simulink model "Integrated_Model"  (R2018a)
settings: Solver=VariableStepAuto  StartTime=0.0  StopTime=500  RelTol=1e-3
undefined symbols (not defined in the file or in its folder): sgn
libraries: simulink x5
settings Model: Creator=梁鑫  LastModifiedBy=梁鑫

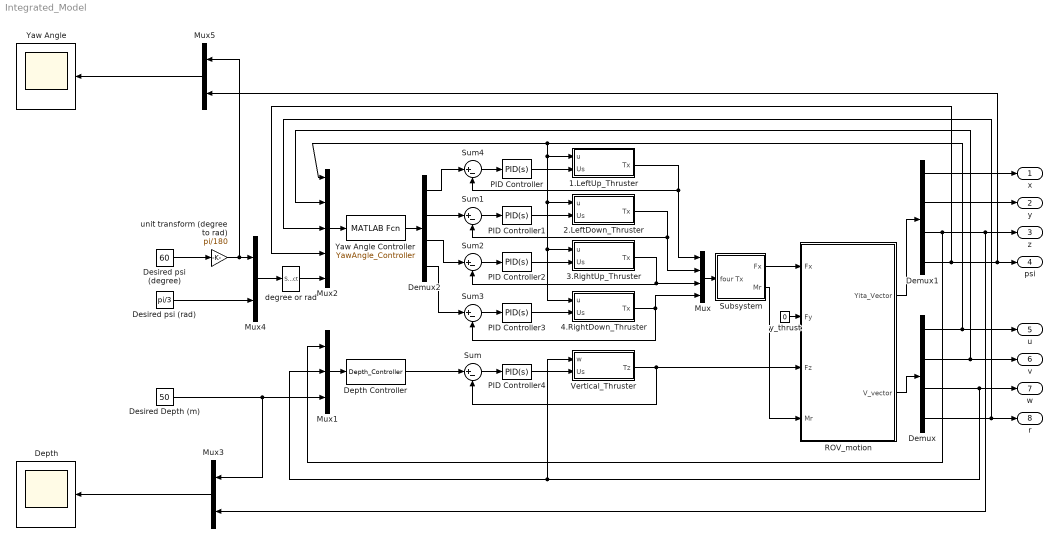
== system Integrated_Model ==
  1.LeftUp_Thruster : Subsystem
  2.LeftDown_Thruster : Subsystem
  3.RightUp_Thruster : Subsystem
  4.RightDown_Thruster : Subsystem
  Demux : Demux
  Demux1 : Demux
  Demux2 : Demux
  Depth : Scope
  Depth Controller : MATLABFcn  MATLABFcn=Depth_Controller  OutputDimensions=1
  Desired Depth (m) : Constant  Value=50
  Desired psi (rad) : Constant  Value=pi/3
  Desired psi (degree) : Constant  Value=60
  Mux : Mux
  Mux1 : Mux  Inputs=3
  Mux2 : Mux  Inputs=5
  Mux3 : Mux  Inputs=2
  Mux4 : Mux  Inputs=2
  Mux5 : Mux  Inputs=2
  PID Controller{,1..3} (4 alike) : simulink/Continuous/PID Controller  Controller=PID  TimeDomain=Continuous-time  SampleTime=-1  IntegratorMethod=Forward Euler  FilterMethod=Forward Euler  Form=Parallel  UseFilter=on  ControllerParametersSource=internal  P=1  I=5  D=0  N=100  InitialConditionSource=internal  InitialConditionForIntegrator=0  InitialConditionForFilter=0  ExternalReset=none  LimitOutput=off  UpperSaturationLimit=inf  LowerSaturationLimit=-inf  LinearizeAsGain=on  AntiWindupMode=none  Kb=1  TrackingMode=off  Kt=1  PParamMin=[]  PParamMax=[]  IParamMin=[]  IParamMax=[]  DParamMin=[]  DParamMax=[]  NParamMin=[]  NParamMax=[]  KbParamMin=[]  KbParamMax=[]  KtParamMin=[]  KtParamMax=[]  POutMin=[]  POutMax=[]  IOutMin=[]  IOutMax=[]  DOutMin=[]  DOutMax=[]  NOutMin=[]  NOutMax=[]  KbOutMin=[]  KbOutMax=[]  KtOutMin=[]  KtOutMax=[]  IntegratorOutMin=[]  IntegratorOutMax=[]  FilterOutMin=[]  FilterOutMax=[]  SumOutMin=[]  SumOutMax=[]  SumI1OutMin=[]  SumI1OutMax=[]  SumI2OutMin=[]  SumI2OutMax=[]  SumI3OutMin=[]  SumI3OutMax=[]  SumDOutMin=[]  SumDOutMax=[]  SaturationOutMin=[]  SaturationOutMax=[]  IntegratorContinuousStateAttributes=''  IntegratorStateMustResolveToSignalObject=off  IntegratorRTWStateStorageClass=Auto  FilterContinuousStateAttributes=''  FilterStateMustResolveToSignalObject=off  FilterRTWStateStorageClass=Auto  DifferentiatorICPrevScaledInput=0  DifferentiatorOutMin=[]  DifferentiatorOutMax=[]  FilterDiffOutCoefMin=[]  FilterDiffOutCoefMax=[]  SumDenOutMin=[]  SumDenOutMax=[]  SumNumOutMin=[]  SumNumOutMax=[]  ReciprocalOutMin=[]  ReciprocalOutMax=[]  DivideOutMin=[]  DivideOutMax=[]  TunerSelectOption=Transfer Function Based (PID Tuner App)
  PID Controller4 : simulink/Continuous/PID Controller  Controller=PID  TimeDomain=Continuous-time  SampleTime=-1  IntegratorMethod=Forward Euler  FilterMethod=Forward Euler  Form=Parallel  UseFilter=on  ControllerParametersSource=internal  P=1  I=5  D=1  N=100  InitialConditionSource=internal  InitialConditionForIntegrator=0  InitialConditionForFilter=0  ExternalReset=none  LimitOutput=off  UpperSaturationLimit=inf  LowerSaturationLimit=-inf  LinearizeAsGain=on  AntiWindupMode=none  Kb=1  TrackingMode=off  Kt=1  PParamMin=[]  PParamMax=[]  IParamMin=[]  IParamMax=[]  DParamMin=[]  DParamMax=[]  NParamMin=[]  NParamMax=[]  KbParamMin=[]  KbParamMax=[]  KtParamMin=[]  KtParamMax=[]  POutMin=[]  POutMax=[]  IOutMin=[]  IOutMax=[]  DOutMin=[]  DOutMax=[]  NOutMin=[]  NOutMax=[]  KbOutMin=[]  KbOutMax=[]  KtOutMin=[]  KtOutMax=[]  IntegratorOutMin=[]  IntegratorOutMax=[]  FilterOutMin=[]  FilterOutMax=[]  SumOutMin=[]  SumOutMax=[]  SumI1OutMin=[]  SumI1OutMax=[]  SumI2OutMin=[]  SumI2OutMax=[]  SumI3OutMin=[]  SumI3OutMax=[]  SumDOutMin=[]  SumDOutMax=[]  SaturationOutMin=[]  SaturationOutMax=[]  IntegratorContinuousStateAttributes=''  IntegratorStateMustResolveToSignalObject=off  IntegratorRTWStateStorageClass=Auto  FilterContinuousStateAttributes=''  FilterStateMustResolveToSignalObject=off  FilterRTWStateStorageClass=Auto  DifferentiatorICPrevScaledInput=0  DifferentiatorOutMin=[]  DifferentiatorOutMax=[]  FilterDiffOutCoefMin=[]  FilterDiffOutCoefMax=[]  SumDenOutMin=[]  SumDenOutMax=[]  SumNumOutMin=[]  SumNumOutMax=[]  ReciprocalOutMin=[]  ReciprocalOutMax=[]  DivideOutMin=[]  DivideOutMax=[]  TunerSelectOption=Transfer Function Based (PID Tuner App)
  ROV_motion : Subsystem
  Subsystem : Subsystem
  Sum{,1..4} (5 alike) : Sum  Inputs=|+-
  Vertical_Thruster : Subsystem
  Yaw Angle : Scope
  Yaw Angle Controller : MATLABFcn  MATLABFcn=YawAngle_Controller  OutputDimensions=4
  degree or rad : Selector  InputPortWidth=2  IndexOptions=Index vector (dialog)  Indices=1  OutputSizes=1
  unit transform (degree to rad) : Gain  Gain=pi/180
  y_thrust : Constant  Value=0
  x : Outport
  y : Outport  Port=2
  z : Outport  Port=3
  psi : Outport  Port=4
  u : Outport  Port=5
  v : Outport  Port=6
  w : Outport  Port=7
  r : Outport  Port=8
  wires:
  y_thrust/1 -> ROV_motion/2(Fy)
  Demux1/3 -> Mux1/1, Mux3/2, z/1
  Demux1/4 -> Mux5/2, psi/1, Mux2/4
  ROV_motion/2(V_vector) -> Demux/1
  Demux/2 -> Mux2/2, v/1
  Demux/3 -> Mux1/2, Vertical_Thruster/1(w), w/1
  Demux/4 -> Mux2/3, r/1
  Demux/1 -> Mux2/1, 4.RightDown_Thruster/1(u), 3.RightUp_Thruster/1(u), 2.LeftDown_Thruster/1(u), 1.LeftUp_Thruster/1(u), u/1
  Subsystem/1(Fx) -> ROV_motion/1(Fx)
  Subsystem/2(Mr) -> ROV_motion/4(Mr)
  1.LeftUp_Thruster/1(Tx) -> Sum4/2, Mux/1
  2.LeftDown_Thruster/1(Tx) -> Sum1/2, Mux/2
  3.RightUp_Thruster/1(Tx) -> Sum2/2, Mux/3
  4.RightDown_Thruster/1(Tx) -> Sum3/2, Mux/4
  Mux/1 -> Subsystem/1(four Tx)
  PID Controller/1 -> 1.LeftUp_Thruster/2(Us)
  Sum4/1 -> PID Controller/1
  Sum1/1 -> PID Controller1/1
  Sum2/1 -> PID Controller2/1
  Sum3/1 -> PID Controller3/1
  PID Controller3/1 -> 4.RightDown_Thruster/2(Us)
  PID Controller2/1 -> 3.RightUp_Thruster/2(Us)
  PID Controller1/1 -> 2.LeftDown_Thruster/2(Us)
  Vertical_Thruster/1(Tz) -> Sum/2, ROV_motion/3(Fz)
  Mux4/1 -> degree or rad/1
  Yaw Angle Controller/1 -> Demux2/1
  Mux2/1 -> Yaw Angle Controller/1
  Desired psi (rad)/1 -> Mux4/2
  unit transform (degree to rad)/1 -> Mux5/1, Mux4/1
  degree or rad/1 -> Mux2/5
  Demux2/1 -> Sum4/1
  Demux2/2 -> Sum1/1
  Demux2/3 -> Sum2/1
  Demux2/4 -> Sum3/1
  Sum/1 -> PID Controller4/1
  Depth Controller/1 -> Sum/1
  Mux1/1 -> Depth Controller/1
  PID Controller4/1 -> Vertical_Thruster/2(Us)
  Desired Depth (m)/1 -> Mux3/1, Mux1/3
  ROV_motion/1(Yita_Vector) -> Demux1/1
  Demux1/1 -> x/1
  Demux1/2 -> y/1
  Desired psi (degree)/1 -> unit transform (degree to rad)/1
  Mux3/1 -> Depth/1
  Mux5/1 -> Yaw Angle/1

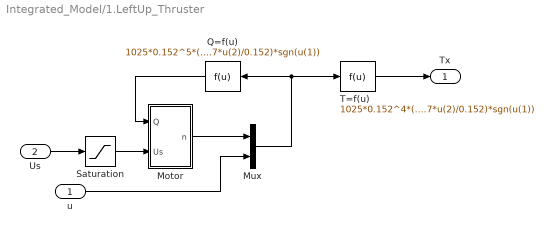
== system Integrated_Model/1.LeftUp_Thruster ==
  u : Inport
  Us : Inport  Port=2
  Motor : Subsystem
  Mux : Mux  Inputs=2
  Q=f(u) : Fcn  Expr=1025*0.152^5*(0.0271*u(1)^2-0.0157*u(1)*0.7*u(2)/0.152)*sgn(u(1))
  Saturation : Saturate  UpperLimit=100  LowerLimit=-100
  T=f(u) : Fcn  Expr=1025*0.152^4*(0.2299*u(1)^2-0.2251*u(1)*0.7*u(2)/0.152)*sgn(u(1))
  Tx : Outport
  wires:
  Saturation/1 -> Motor/2(Us)
  Mux/1 -> T=f(u)/1, Q=f(u)/1
  Q=f(u)/1 -> Motor/1(Q)
  Motor/1(n) -> Mux/1
  u/1 -> Mux/2
  T=f(u)/1 -> Tx/1
  Us/1 -> Saturation/1

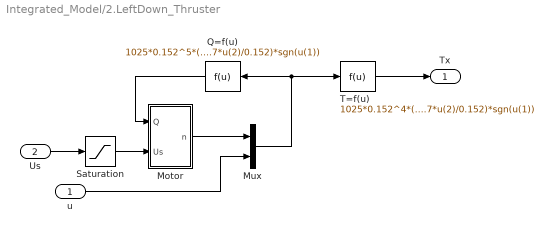
== system Integrated_Model/2.LeftDown_Thruster ==
  u : Inport
  Us : Inport  Port=2
  Motor : Subsystem
  Mux : Mux  Inputs=2
  Q=f(u) : Fcn  Expr=1025*0.152^5*(0.0271*u(1)^2-0.0157*u(1)*0.7*u(2)/0.152)*sgn(u(1))
  Saturation : Saturate  UpperLimit=100  LowerLimit=-100
  T=f(u) : Fcn  Expr=1025*0.152^4*(0.2299*u(1)^2-0.2251*u(1)*0.7*u(2)/0.152)*sgn(u(1))
  Tx : Outport
  wires:
  Us/1 -> Saturation/1
  T=f(u)/1 -> Tx/1
  u/1 -> Mux/2
  Motor/1(n) -> Mux/1
  Q=f(u)/1 -> Motor/1(Q)
  Mux/1 -> Q=f(u)/1, T=f(u)/1
  Saturation/1 -> Motor/2(Us)

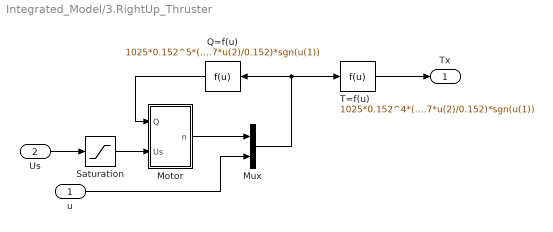
== system Integrated_Model/3.RightUp_Thruster ==
  u : Inport
  Us : Inport  Port=2
  Motor : Subsystem
  Mux : Mux  Inputs=2
  Q=f(u) : Fcn  Expr=1025*0.152^5*(0.0271*u(1)^2-0.0157*u(1)*0.7*u(2)/0.152)*sgn(u(1))
  Saturation : Saturate  UpperLimit=100  LowerLimit=-100
  T=f(u) : Fcn  Expr=1025*0.152^4*(0.2299*u(1)^2-0.2251*u(1)*0.7*u(2)/0.152)*sgn(u(1))
  Tx : Outport
  wires:
  Saturation/1 -> Motor/2(Us)
  Mux/1 -> T=f(u)/1, Q=f(u)/1
  Q=f(u)/1 -> Motor/1(Q)
  Motor/1(n) -> Mux/1
  u/1 -> Mux/2
  T=f(u)/1 -> Tx/1
  Us/1 -> Saturation/1

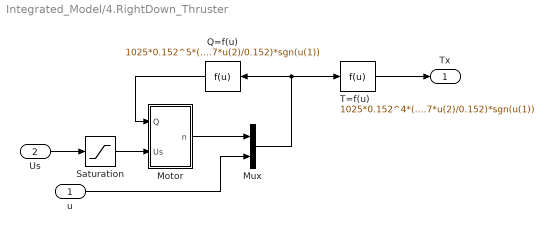
== system Integrated_Model/4.RightDown_Thruster ==
  u : Inport
  Us : Inport  Port=2
  Motor : Subsystem
  Mux : Mux  Inputs=2
  Q=f(u) : Fcn  Expr=1025*0.152^5*(0.0271*u(1)^2-0.0157*u(1)*0.7*u(2)/0.152)*sgn(u(1))
  Saturation : Saturate  UpperLimit=100  LowerLimit=-100
  T=f(u) : Fcn  Expr=1025*0.152^4*(0.2299*u(1)^2-0.2251*u(1)*0.7*u(2)/0.152)*sgn(u(1))
  Tx : Outport
  wires:
  Us/1 -> Saturation/1
  T=f(u)/1 -> Tx/1
  u/1 -> Mux/2
  Motor/1(n) -> Mux/1
  Q=f(u)/1 -> Motor/1(Q)
  Mux/1 -> Q=f(u)/1, T=f(u)/1
  Saturation/1 -> Motor/2(Us)

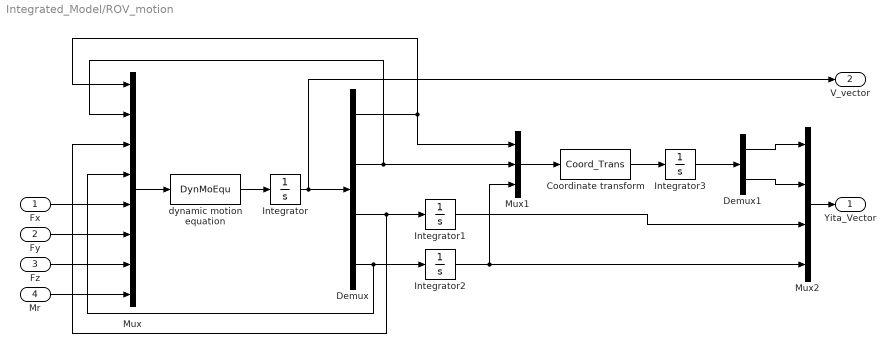
== system Integrated_Model/ROV_motion ==
  Fx : Inport
  Fy : Inport  Port=2
  Fz : Inport  Port=3
  Mr : Inport  Port=4
  Coordinate transform : MATLABFcn  MATLABFcn=Coord_Trans  OutputDimensions=2
  Demux : Demux
  Demux1 : Demux  Outputs=2
  Integrator{,1..3} (4 alike) : Integrator
  Mux : Mux  Inputs=8
  Mux1 : Mux  Inputs=3
  Mux2 : Mux
  dynamic motion equation : MATLABFcn  MATLABFcn=DynMoEqu  OutputDimensions=4
  Yita_Vector : Outport
  V_vector : Outport  Port=2
  wires:
  dynamic motion equation/1 -> Integrator/1
  Demux/4 -> Mux/4, Integrator2/1
  Fx/1 -> Mux/5
  Integrator/1 -> V_vector/1, Demux/1
  Mr/1 -> Mux/8
  Coordinate transform/1 -> Integrator3/1
  Demux/3 -> Mux/3, Integrator1/1
  Mux/1 -> dynamic motion equation/1
  Fz/1 -> Mux/7
  Demux/2 -> Mux/2, Mux1/2
  Mux1/1 -> Coordinate transform/1
  Fy/1 -> Mux/6
  Integrator2/1 -> Mux1/3, Mux2/4
  Demux/1 -> Mux1/1, Mux/1
  Integrator3/1 -> Demux1/1
  Demux1/1 -> Mux2/1
  Demux1/2 -> Mux2/2
  Integrator1/1 -> Mux2/3
  Mux2/1 -> Yita_Vector/1

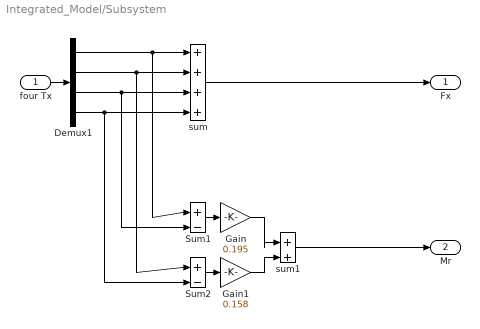
== system Integrated_Model/Subsystem ==
  four Tx : Inport
  Demux1 : Demux
  Gain : Gain  Gain=0.195
  Gain1 : Gain  Gain=0.158
  Sum1 : Sum  Inputs=|+-
  Sum2 : Sum  Inputs=|+-
  sum : Sum  Inputs=++++
  sum1 : Sum  Inputs=|++
  Fx : Outport
  Mr : Outport  Port=2
  wires:
  Sum1/1 -> Gain/1
  Demux1/1 -> Sum1/1, sum/1
  Demux1/4 -> Sum2/2, sum/4
  Gain1/1 -> sum1/2
  Demux1/3 -> Sum1/2, sum/3
  Demux1/2 -> Sum2/1, sum/2
  Gain/1 -> sum1/1
  Sum2/1 -> Gain1/1
  sum/1 -> Fx/1
  sum1/1 -> Mr/1
  four Tx/1 -> Demux1/1

== system Integrated_Model/Vertical_Thruster ==
  w : Inport
  Us : Inport  Port=2
  Motor : Subsystem
  Mux : Mux  Inputs=2
  Q=f(u) : Fcn  Expr=1025*0.152^5*(0.0271*u(1)^2-0.0157*u(1)*0.7*u(2)/0.152)*sgn(u(1))
  Saturation : Saturate  UpperLimit=100  LowerLimit=-100
  T=f(u) : Fcn  Expr=1025*0.152^4*(0.2299*u(1)^2-0.2251*u(1)*0.7*u(2)/0.152)*sgn(u(1))
  Tz : Outport
  wires:
  Saturation/1 -> Motor/2(Us)
  Mux/1 -> T=f(u)/1, Q=f(u)/1
  Q=f(u)/1 -> Motor/1(Q)
  Motor/1(n) -> Mux/1
  w/1 -> Mux/2
  T=f(u)/1 -> Tz/1
  Us/1 -> Saturation/1

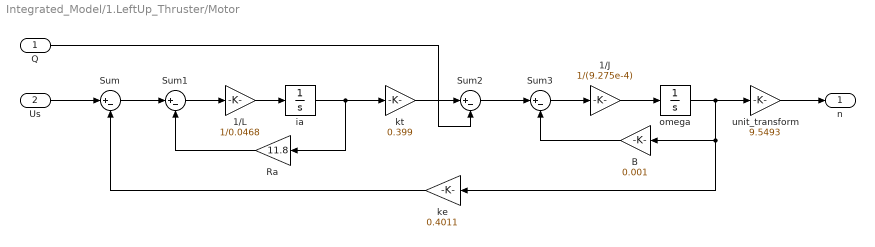
== system Integrated_Model/1.LeftUp_Thruster/Motor ==
  Q : Inport
  Us : Inport  Port=2
  1/J : Gain  Gain=1/(9.275e-4)
  1/L : Gain  Gain=1/0.0468
  B : Gain  Gain=0.001
  Ra : Gain  Gain=11.8
  Sum{,1..3} (4 alike) : Sum  Inputs=|+-
  ia : Integrator
  ke : Gain  Gain=0.4011
  kt : Gain  Gain=0.399
  omega : Integrator
  unit_transform : Gain  Gain=9.5493
  n : Outport
  wires:
  Sum2/1 -> Sum3/1
  Sum1/1 -> 1/L/1
  Sum/1 -> Sum1/1
  ia/1 -> Ra/1, kt/1
  Q/1 -> Sum2/2
  Ra/1 -> Sum1/2
  1/J/1 -> omega/1
  Sum3/1 -> 1/J/1
  Us/1 -> Sum/1
  B/1 -> Sum3/2
  1/L/1 -> ia/1
  omega/1 -> unit_transform/1, ke/1, B/1
  kt/1 -> Sum2/1
  ke/1 -> Sum/2
  unit_transform/1 -> n/1

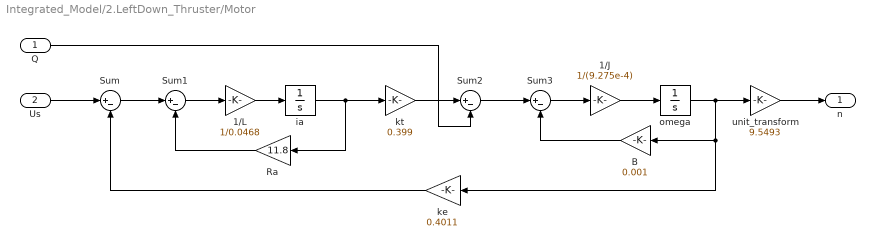
== system Integrated_Model/2.LeftDown_Thruster/Motor ==
  Q : Inport
  Us : Inport  Port=2
  1/J : Gain  Gain=1/(9.275e-4)
  1/L : Gain  Gain=1/0.0468
  B : Gain  Gain=0.001
  Ra : Gain  Gain=11.8
  Sum{,1..3} (4 alike) : Sum  Inputs=|+-
  ia : Integrator
  ke : Gain  Gain=0.4011
  kt : Gain  Gain=0.399
  omega : Integrator
  unit_transform : Gain  Gain=9.5493
  n : Outport
  wires:
  unit_transform/1 -> n/1
  ke/1 -> Sum/2
  kt/1 -> Sum2/1
  omega/1 -> B/1, ke/1, unit_transform/1
  1/L/1 -> ia/1
  B/1 -> Sum3/2
  Us/1 -> Sum/1
  Sum3/1 -> 1/J/1
  1/J/1 -> omega/1
  Ra/1 -> Sum1/2
  Q/1 -> Sum2/2
  ia/1 -> kt/1, Ra/1
  Sum/1 -> Sum1/1
  Sum1/1 -> 1/L/1
  Sum2/1 -> Sum3/1

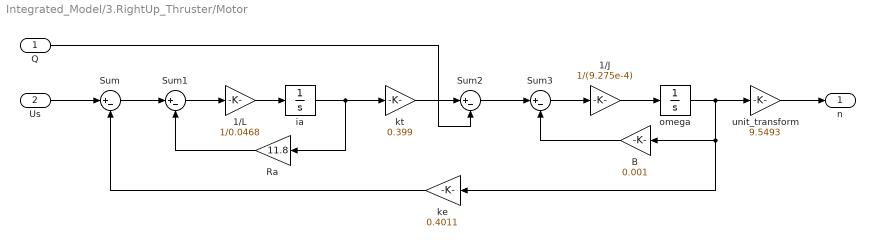
== system Integrated_Model/3.RightUp_Thruster/Motor ==
  Q : Inport
  Us : Inport  Port=2
  1/J : Gain  Gain=1/(9.275e-4)
  1/L : Gain  Gain=1/0.0468
  B : Gain  Gain=0.001
  Ra : Gain  Gain=11.8
  Sum{,1..3} (4 alike) : Sum  Inputs=|+-
  ia : Integrator
  ke : Gain  Gain=0.4011
  kt : Gain  Gain=0.399
  omega : Integrator
  unit_transform : Gain  Gain=9.5493
  n : Outport
  wires:
  Sum2/1 -> Sum3/1
  Sum1/1 -> 1/L/1
  Sum/1 -> Sum1/1
  ia/1 -> Ra/1, kt/1
  Q/1 -> Sum2/2
  Ra/1 -> Sum1/2
  1/J/1 -> omega/1
  Sum3/1 -> 1/J/1
  Us/1 -> Sum/1
  B/1 -> Sum3/2
  1/L/1 -> ia/1
  omega/1 -> unit_transform/1, ke/1, B/1
  kt/1 -> Sum2/1
  ke/1 -> Sum/2
  unit_transform/1 -> n/1

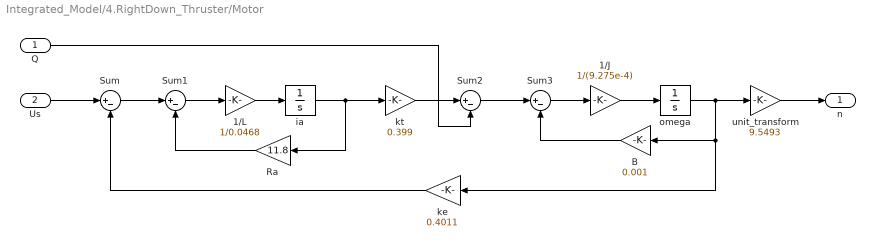
== system Integrated_Model/4.RightDown_Thruster/Motor ==
  Q : Inport
  Us : Inport  Port=2
  1/J : Gain  Gain=1/(9.275e-4)
  1/L : Gain  Gain=1/0.0468
  B : Gain  Gain=0.001
  Ra : Gain  Gain=11.8
  Sum{,1..3} (4 alike) : Sum  Inputs=|+-
  ia : Integrator
  ke : Gain  Gain=0.4011
  kt : Gain  Gain=0.399
  omega : Integrator
  unit_transform : Gain  Gain=9.5493
  n : Outport
  wires:
  unit_transform/1 -> n/1
  ke/1 -> Sum/2
  kt/1 -> Sum2/1
  omega/1 -> B/1, ke/1, unit_transform/1
  1/L/1 -> ia/1
  B/1 -> Sum3/2
  Us/1 -> Sum/1
  Sum3/1 -> 1/J/1
  1/J/1 -> omega/1
  Ra/1 -> Sum1/2
  Q/1 -> Sum2/2
  ia/1 -> kt/1, Ra/1
  Sum/1 -> Sum1/1
  Sum1/1 -> 1/L/1
  Sum2/1 -> Sum3/1

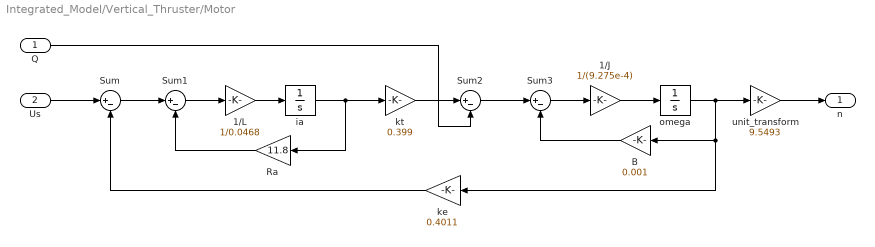
== system Integrated_Model/Vertical_Thruster/Motor ==
  Q : Inport
  Us : Inport  Port=2
  1/J : Gain  Gain=1/(9.275e-4)
  1/L : Gain  Gain=1/0.0468
  B : Gain  Gain=0.001
  Ra : Gain  Gain=11.8
  Sum{,1..3} (4 alike) : Sum  Inputs=|+-
  ia : Integrator
  ke : Gain  Gain=0.4011
  kt : Gain  Gain=0.399
  omega : Integrator
  unit_transform : Gain  Gain=9.5493
  n : Outport
  wires:
  Sum2/1 -> Sum3/1
  Sum1/1 -> 1/L/1
  Sum/1 -> Sum1/1
  ia/1 -> Ra/1, kt/1
  Q/1 -> Sum2/2
  Ra/1 -> Sum1/2
  1/J/1 -> omega/1
  Sum3/1 -> 1/J/1
  Us/1 -> Sum/1
  B/1 -> Sum3/2
  1/L/1 -> ia/1
  omega/1 -> unit_transform/1, ke/1, B/1
  kt/1 -> Sum2/1
  ke/1 -> Sum/2
  unit_transform/1 -> n/1
